simulink model "ExternalSources"  (Simulink 6.4)
settings: Solver=FixedStepDiscrete  SolverMode=SingleTasking  StartTime=0  StopTime=10  FixedStep=0.001  RelTol=1e-3
libraries: ecrobot_nxt_lib x4
settings Model: Creator=tchikama  LastModifiedBy=tchikama  ProdHWDeviceType=ARM7
settings DataIOCC: SaveOutput=off  SignalLogging=off  SaveTime=off
settings OptimizationCC: InlineParams=on  InlineInvariantSignals=on  RollThreshold=2  StateBitsets=on  DataBitsets=on  UseTempVars=on  InitFltsAndDblsToZero=off  NoFixptDivByZeroProtection=on  EfficientFloat2IntCast=on  OptimizeModelRefInitCode=on  LifeSpan=1
settings DebuggingCC: ConsistencyChecking=warning  SignalInfNanChecking=warning  ReadBeforeWriteMsg=DisableAll  WriteAfterWriteMsg=DisableAll  WriteAfterReadMsg=DisableAll  AlgebraicLoopMsg=error  CheckExecutionContextPreStartOutputMsg=on  CheckExecutionContextRuntimeOutputMsg=on  SolverPrmCheckMsg=none  SingleTaskRateTransMsg=warning  TasksWithSamePriorityMsg=none  IntegerOverflowMsg=error  ParameterPrecisionLossMsg=none  UnconnectedInputMsg=error  UnconnectedOutputMsg=error  UnconnectedLineMsg=error  UniqueDataStoreMsg=error  BusObjectLabelMismatch=error  RootOutportRequireBusObject=error  ModelReferenceIOMsg=warning  ModelReferenceVersionMismatchMessage=warning  ModelReferenceIOMismatchMessage=warning
settings HardwareCC: ProdIntDivRoundTo=Zero  ProdEndianess=LittleEndian  ProdHWDeviceType=ARM7  TargetHWDeviceType=32-bit Generic
settings ModelReferenceCC: ModelReferenceNumInstancesAllowed=Single
settings RTWCC: SystemTargetFile=ert.tlc  GenCodeOnly=on  GenerateMakefile=off  TemplateMakefile=ert_default_tmf  Description=Real-Time Workshop Embedded Coder (no auto configuration)  GenerateReport=on  RTWVerbose=off  ProcessScript=ert_make_rtw_hook  IncludeHyperlinkInReport=on  LaunchReport=on
settings CodeAppCC: ForceParamTrailComments=on  IgnoreCustomStorageClasses=off  SFDataObjDesc=on  PrefixModelToSubsysFcnNames=off  CustomSymbolStrGlobalVar=rt$N$M  CustomSymbolStrType=$N$M  CustomSymbolStrFcn=$N$M$F  CustomSymbolStrMacro=$N$M  InsertBlockDesc=on
settings ERTTargetCC: TargetFcnLib=ansi_tfl_tmw.mat  GenFloatMathFcnCalls=GNU  IncludeMdlTerminateFcn=off  SuppressErrorStatus=on  IncludeERTFirstTime=on  SupportAbsoluteTime=off  SupportNonFinite=off  SupportComplex=off  PurelyIntegerCode=on  InlinedParameterPlacement=NonHierarchical  RootIOFormat=Structure reference  ERTCustomFileTemplate=example_file_process.tlc  InitialValueSource=Model

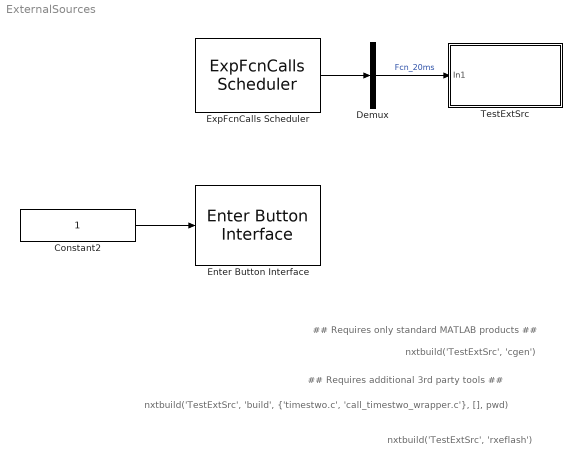
== system ExternalSources ==
  note: nxtbuild('TestExtSrc', 'build', {'timestwo.c', 'call_timestwo_wrapper.c'}, [], pwd)
  note: nxtbuild('TestExtSrc', 'rxeflash')
  note: nxtbuild('TestExtSrc', 'cgen')
  note: ## Requires only standard MATLAB products ##
  note: ## Requires additional 3rd party tools ##
  Constant2 : Constant  Value=1  OutDataType=sfix(16)  ConRadixGroup=Use specified scaling  OutScaling=2^0  SampleTime=inf  FramePeriod=inf
  Demux : Demux  Outputs=1
  Enter Button Interface : ecrobot_nxt_lib/Enter Button Interface  SystemSampleTime=-1
  ExpFcnCalls Scheduler : ecrobot_nxt_lib/ExpFcnCalls Scheduler  fcname='Fcn_20ms'  fctrigger=[20]  ts=0.001  platform=OSEK  stacksize=[512]  bd_mode=Slave
  TestExtSrc : Subsystem
  wires:
  ExpFcnCalls Scheduler/1 -> Demux/1
  Demux/1 -> TestExtSrc/1(In1)  "Fcn_20ms"
  Constant2/1 -> Enter Button Interface/1

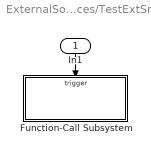
== system ExternalSources/TestExtSrc ==
  In1 : Inport  Orientation=down
  Function-Call Subsystem : Subsystem  TreatAsAtomicUnit=on
  wires:
  In1/1 -> Function-Call Subsystem/Trigger

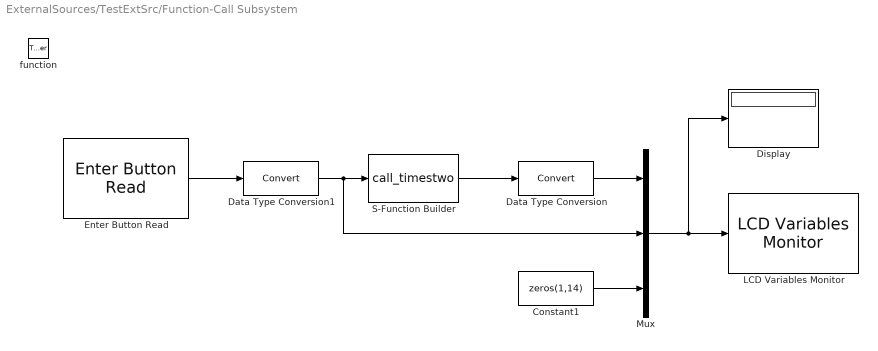
== system ExternalSources/TestExtSrc/Function-Call Subsystem ==
  function : TriggerPort  TriggerType=function-call
  Constant1 : Constant  Value=zeros(1,14)  OutDataTypeMode=int32  OutDataType=sfix(16)  ConRadixGroup=Use specified scaling  OutScaling=2^0  SampleTime=inf  FramePeriod=inf
  Data Type Conversion : DataTypeConversion  OutDataTypeMode=int32
  Data Type Conversion1 : DataTypeConversion  OutDataTypeMode=int32
  Display : Display
  Enter Button Read : ecrobot_nxt_lib/Enter Button Read  SystemSampleTime=-1
  LCD Variables Monitor : ecrobot_nxt_lib/LCD Variables Monitor
  Mux : Mux  Inputs=3
  S-Function Builder : S-Function  InitFcn=try, set_param(gcb,'FunctionName','call_timestwo'), end  FunctionName=call_timestwo  SFunctionModules=call_timestwo_wrapper timestwo  WizardData=DataTag0  mask(S-Function Builder){}
      mask init:
      | val = [[.9  0.75 0.75 1 1 .9 .9 1]',[1 1 0.75 0.75 .9 .9 1 .9]'];try , sys = get_param(gcb,'SfunBuilderFcnName');if isempty(sys), sys = get_param(gcb,'FunctionName'); end,catch, sys = get_param(gcb,'FunctionName'); end
      settings: CopyFcn=set_param(gcbh,'LinkStatus','none')  PreSaveFcn=try, set_param(gcb,'FunctionName','call_timestwo'), end  OpenFcn=sfunctionwizard(gcbh)
      mask Display: plot(val(:,1),val(:,2)),disp(sys)port_label('input',1,'u0')port_label('output',1,'y0')
  wires:
  Data Type Conversion/1 -> Mux/1
  Mux/1 -> LCD Variables Monitor/1, Display/1
  Enter Button Read/1 -> Data Type Conversion1/1
  Constant1/1 -> Mux/3
  Data Type Conversion1/1 -> Mux/2, S-Function Builder/1
  S-Function Builder/1 -> Data Type Conversion/1
